simulink model "Model_Composite_2Link_NN_highgain"  (R2019a)
settings: Solver=ode45  StartTime=0.0  StopTime=25  FixedStep=0.0001  RelTol=1e-6  EnableMultiTasking=on
values from neighbouring files (symbols this model uses):
  alpha = 10    [Sim6_highgain.m]
  k = 50    [Sim6_highgain.m]
  kn = 10    [Sim6_highgain.m]
  ks = 1    [Sim6_highgain.m]
  proj1 = 4.5    [Sim6_highgain.m]
  proj2 = 6.7    [Sim6_highgain.m]
  v_initial = zeros(7,5)    [Sim6_highgain.m]
  w_initial = zeros(6,2)    [Sim6_highgain.m]
undefined symbols (not defined in the file or in its folder): gamma1, gamma2
settings Model: Creator=Tenghu  LastModifiedBy=normal
settings DataIOCC: SaveFormat=Array  SignalLoggingSaveFormat=ModelDataLogs  ReturnWorkspaceOutputs=off
settings OptimizationCC: ExpressionDepthLimit=2147483647  EfficientMapNaN2IntZero=off  LifeSpan=inf
settings DebuggingCC: UnderspecifiedInitializationDetection=Classic  MergeDetectMultiDrivingBlocksExec=none  FcnCallInpInsideContextMsg=warning  StateNameClashWarn=warning  SFUnexpectedBacktrackingDiag=warning  SFNoUnconditionalDefaultTransitionDiag=warning  SFExecutionAtInitializationDiag=none  ArithmeticOperatorsInVariantConditions=warning
settings HardwareCC: ProdBitPerPointer=32  ProdBitPerSizeT=32  ProdBitPerPtrDiffT=32  ProdLargestAtomicFloat=None  ProdIntDivRoundTo=Undefined  ProdEndianess=Unspecified  ProdWordSize=32  ProdHWDeviceType=32-bit Generic  TargetBitPerPointer=64  TargetBitPerSizeT=64  TargetBitPerPtrDiffT=64  TargetLongLongMode=on  TargetIntDivRoundTo=Zero  TargetEndianess=LittleEndian  TargetWordSize=64  TargetHWDeviceType=MATLAB Host  ProdEqTarget=off
settings ModelReferenceCC: PropagateSignalLabelsOutOfModel=off
settings SFSimCC: SimUseLocalCustomCode=off  SimParseCustomCode=off
settings RTWCC: RTWUseLocalCustomCode=off
settings CodeAppCC: MaxIdLength=128  StateflowObjectComments=on
settings GRTTargetCC: TargetLangStandard=C89/C90 (ANSI)  GeneratePreprocessorConditionals=Disable all  CombineOutputUpdateFcns=off  GRTInterface=on
settings ConfigComp: CovMetricSettings=dw  CovHtmlReporting=on  CovSaveCumulativeToWorkspaceVar=on  CovSaveSingleToWorkspaceVar=on  CovExternalEMLEnable=off

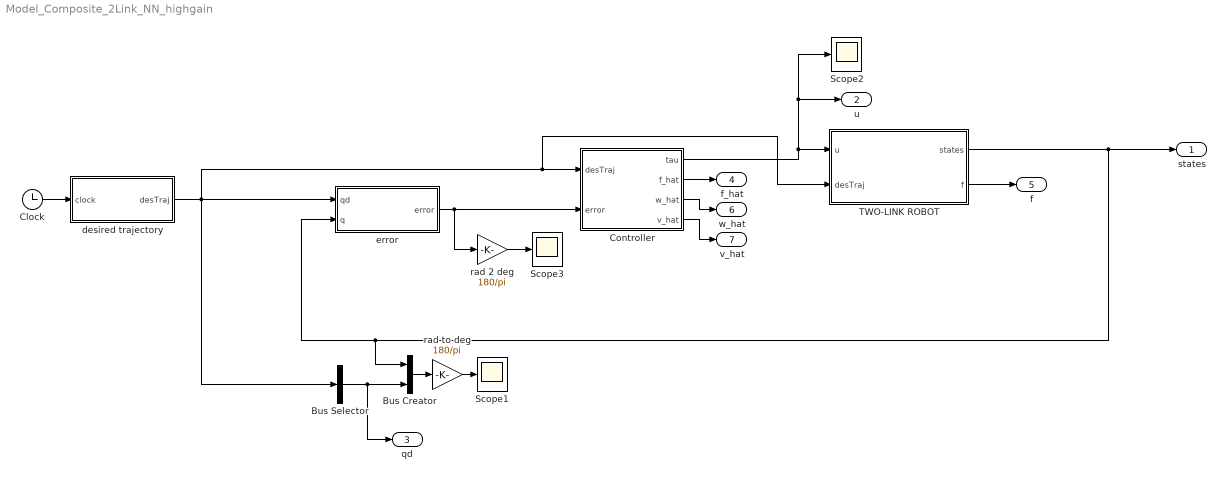
== system Model_Composite_2Link_NN_highgain ==
  Bus Creator : BusCreator  Inputs=2
  Bus Selector : BusSelector  OutputSignals=qd,qdDot  OutputAsBus=on
  Clock : Clock
  Controller : Subsystem
  Scope1 : Scope
  Scope2 : Scope
  Scope3 : Scope
  TWO-LINK ROBOT : Subsystem
  desired trajectory : Subsystem
  error : Subsystem
  rad 2 deg : Gain  Gain=180/pi
  rad to deg : Gain  Gain=180/pi
  states : Outport
  u : Outport  Port=2
  qd : Outport  Port=3
  f_hat : Outport  Port=4
  f : Outport  Port=5
  w_hat : Outport  Port=6
  v_hat : Outport  Port=7
  wires:
  Clock/1 -> desired trajectory/1(clock)
  desired trajectory/1(desTraj) -> error/1(qd), TWO-LINK ROBOT/2(desTraj), Controller/1(desTraj), Bus Selector/1
  rad 2 deg/1 -> Scope3/1
  Bus Creator/1 -> rad to deg/1
  rad to deg/1 -> Scope1/1
  error/1(error) -> Controller/2(error), rad 2 deg/1
  TWO-LINK ROBOT/1(states) -> Bus Creator/1, error/2(q), states/1
  Bus Selector/1 -> qd/1, Bus Creator/2
  Controller/1(tau) -> Scope2/1, u/1, TWO-LINK ROBOT/1(u)
  Controller/2(f_hat) -> f_hat/1
  TWO-LINK ROBOT/2(f) -> f/1
  Controller/3(w_hat) -> w_hat/1
  Controller/4(v_hat) -> v_hat/1

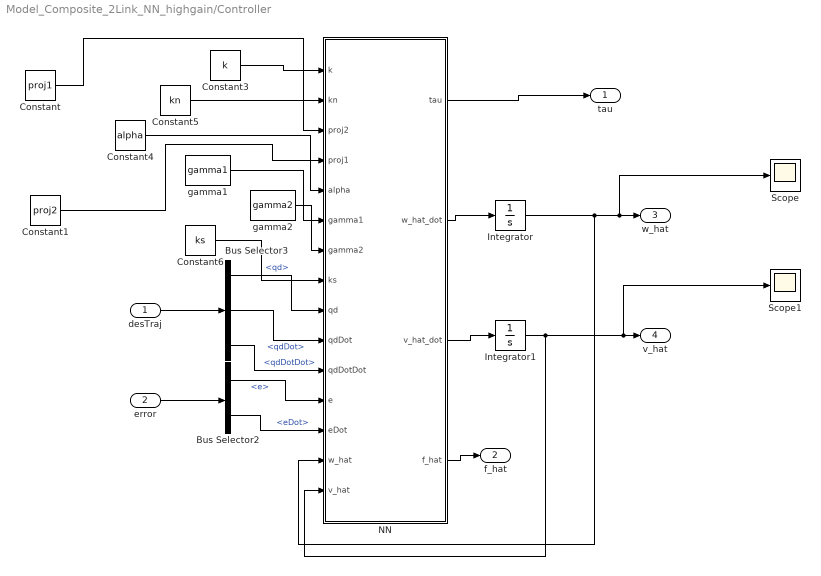
== system Model_Composite_2Link_NN_highgain/Controller ==
  desTraj : Inport
  error : Inport  Port=2
  Bus Selector2 : BusSelector  OutputSignals=e,eDot
  Bus Selector3 : BusSelector  OutputSignals=qd,qdDot,qdDotDot
  Constant : Constant  Value=proj1
  Constant1 : Constant  Value=proj2
  Constant3 : Constant  Value=k
  Constant4 : Constant  Value=alpha
  Constant5 : Constant  Value=kn
  Constant6 : Constant  Value=ks
  Integrator : Integrator  InitialCondition=w_initial
  Integrator1 : Integrator  InitialCondition=v_initial
  NN : MATLAB Function  TreatAsAtomicUnit=on
  Scope : Scope
  Scope1 : Scope
  gamma1 : Constant  Value=gamma1
  gamma2 : Constant  Value=gamma2
  tau : Outport
  f_hat : Outport  Port=2
  w_hat : Outport  Port=3
  v_hat : Outport  Port=4
  wires:
  Bus Selector2/1 -> NN/12(e)  "<e>"
  Bus Selector2/2 -> NN/13(eDot)  "<eDot>"
  error/1 -> Bus Selector2/1
  Bus Selector3/1 -> NN/9(qd)  "<qd>"
  Bus Selector3/3 -> NN/11(qdDotDot)  "<qdDotDot>"
  desTraj/1 -> Bus Selector3/1
  Bus Selector3/2 -> NN/10(qdDot)  "<qdDot>"
  Constant3/1 -> NN/1(k)
  Constant4/1 -> NN/5(alpha)
  Constant5/1 -> NN/2(kn)
  NN/2(w_hat_dot) -> Integrator/1
  NN/3(v_hat_dot) -> Integrator1/1
  Integrator1/1 -> Scope1/1, v_hat/1, NN/15(v_hat)
  Integrator/1 -> Scope/1, w_hat/1, NN/14(w_hat)
  gamma1/1 -> NN/6(gamma1)
  gamma2/1 -> NN/7(gamma2)
  NN/1(tau) -> tau/1
  NN/4(f_hat) -> f_hat/1
  Constant6/1 -> NN/8(ks)
  Constant/1 -> NN/3(proj2)
  Constant1/1 -> NN/4(proj1)

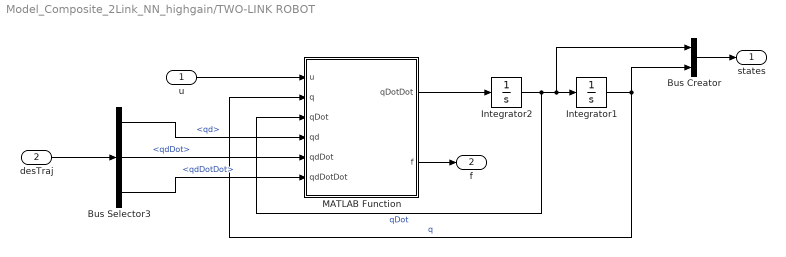
== system Model_Composite_2Link_NN_highgain/TWO-LINK ROBOT ==
  u : Inport
  desTraj : Inport  Port=2
  Bus Creator : BusCreator  Inputs=2
  Bus Selector3 : BusSelector  OutputSignals=qd,qdDot,qdDotDot
  Integrator1 : Integrator  InitialCondition=[0;2]
  Integrator2 : Integrator  InitialCondition=[0;0]
  MATLAB Function : MATLAB Function  TreatAsAtomicUnit=on
  states : Outport
  f : Outport  Port=2
  wires:
  u/1 -> MATLAB Function/1(u)
  Integrator1/1 -> Bus Creator/2, MATLAB Function/2(q)  "q"
  Integrator2/1 -> MATLAB Function/3(qDot), Bus Creator/1, Integrator1/1  "qDot"
  Bus Creator/1 -> states/1
  MATLAB Function/1(qDotDot) -> Integrator2/1
  Bus Selector3/1 -> MATLAB Function/4(qd)  "<qd>"
  Bus Selector3/3 -> MATLAB Function/6(qdDotDot)  "<qdDotDot>"
  desTraj/1 -> Bus Selector3/1
  Bus Selector3/2 -> MATLAB Function/5(qdDot)  "<qdDot>"
  MATLAB Function/2(f) -> f/1

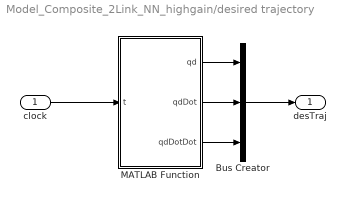
== system Model_Composite_2Link_NN_highgain/desired trajectory ==
  clock : Inport
  Bus Creator : BusCreator  Inputs=3
  MATLAB Function : MATLAB Function  TreatAsAtomicUnit=on
  desTraj : Outport
  wires:
  clock/1 -> MATLAB Function/1(t)
  MATLAB Function/1(qd) -> Bus Creator/1
  MATLAB Function/2(qdDot) -> Bus Creator/2
  MATLAB Function/3(qdDotDot) -> Bus Creator/3
  Bus Creator/1 -> desTraj/1

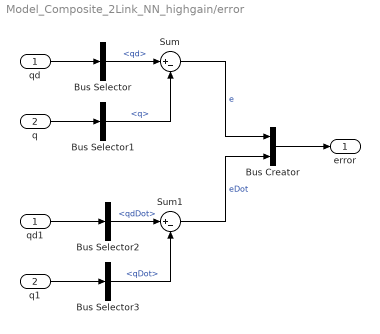
== system Model_Composite_2Link_NN_highgain/error ==
  qd : Inport
  q : Inport  Port=2
  Bus Creator : BusCreator  Inputs=2
  Bus Selector : BusSelector  OutputSignals=qd
  Bus Selector1 : BusSelector  OutputSignals=q
  Bus Selector2 : BusSelector  OutputSignals=qdDot
  Bus Selector3 : BusSelector  OutputSignals=qDot
  Sum : Sum  Inputs=|+-
  Sum1 : Sum  Inputs=|+-
  q1 : InportShadow  Port=2
  qd1 : InportShadow
  error : Outport
  wires:
  qd/1 -> Bus Selector/1
  q/1 -> Bus Selector1/1
  qd1/1 -> Bus Selector2/1
  q1/1 -> Bus Selector3/1
  Bus Selector/1 -> Sum/1  "<qd>"
  Bus Selector1/1 -> Sum/2  "<q>"
  Sum/1 -> Bus Creator/1  "e"
  Bus Selector2/1 -> Sum1/1  "<qdDot>"
  Bus Selector3/1 -> Sum1/2  "<qDot>"
  Bus Creator/1 -> error/1
  Sum1/1 -> Bus Creator/2  "eDot"

== matlab function Model_Composite_2Link_NN_highgain/desired trajectory/MATLAB Function ==
  data: t input; qd output; qdDot output; qdDotDot output
function [qd,qdDot,qdDotDot]  = des_trajectory(t)
%#codegen

% This block supports an embeddable subset of the MATLAB language.
% See the help menu for details. 

qd1=cos(0.5*t);
qd2=2*cos(t);

qd1_dot=-0.5*sin(0.5*t);
qd2_dot=-2*sin(t);

qd1_dotDot = -0.25*cos(0.25*t);
qd2_dotDot = -2*cos(t);

qd=[qd1;qd2];
qdDot = [qd1_dot;qd2_dot];
qdDotDot = [qd1_dotDot; qd2_dotDot];

end

== matlab function Model_Composite_2Link_NN_highgain/Controller/NN ==
  data: k input; kn input; proj2 input; proj1 input; tau output; alpha input; gamma1 input; gamma2 input; ks input; qd input; qdDot input; qdDotDot input; e input; eDot input; w_hat input; v_hat input; w_hat_dot output; v_hat_dot output; f_hat output
function [tau,w_hat_dot,v_hat_dot,f_hat]= controller1(k,kn,proj2, proj1, alpha,gamma1,gamma2,ks,qd,qdDot,qdDotDot,e,eDot,w_hat,v_hat)
%#codegen

q = qd-e; % Check
qDot = qdDot-eDot; % Check
r = eDot+alpha*e; % Check

qd_vec = [1 qd' qdDot' qdDotDot']'; % (7x1)
vq = v_hat'*qd_vec; % (5x7)(7x1) = (5x1)

sigma = exp(-(vq).^2./2); % (5x1)

sigma_vec = [1 sigma']';   % (6x1)
sigma_prime_vec = [1 1 1 1 1; exp(-(vq.^2)./2)*vq'];     %; sigma_prime'; sigma_prime'; sigma_prime'; sigma_prime'; sigma_prime']; % (6x5)

tau = k*r + kn*r + e + w_hat'*sigma_vec ; % (2x6)(6x1)=(2x1)

w_hat_dot = gamma1*sigma_vec*r'; %(6x1)(1x2)=(6x2)
v_hat_dot = gamma2*qd_vec*r'*w_hat'*sigma_prime_vec; %(7x1)(1x2)(2x6)(6x5)=(7x5)

f_hat = w_hat'*sigma_vec; %(2x6)(6x1)=(2x1)

%saturating using projection function
%vHat projection
[v_hat_dot] = Proj(v_hat,v_hat_dot,proj1,-proj1,0.0001);

%w_hat_dot projection function
[w_hat_dot] = Proj(w_hat,w_hat_dot,proj2,-proj2,0.0001);


f_hat = w_hat'*sigma_vec; %(2x6)(6x1)=(2x1)



%projection function definition
function [out] = Proj(theta_hat_curr, theta_hat_dot, upperlim, lowerlim,dt) %functio
[I,J] = size(theta_hat_curr); %initialy matrix definition
out = zeros(I,J);             %initial dummy matrix to be edited later
theta_hat = theta_hat_curr + dt*theta_hat_dot; %proposed update 

% check the proposed update for each index and don't allow it to change
% if it will drive the estimate out of the upper or lower limit
for i = 1:I
    for j = 1:J
        if theta_hat(i,j) >= upperlim && theta_hat_dot(i,j) > 0
            out(i,j) = 0;
        elseif theta_hat(i,j) <= lowerlim && theta_hat_dot(i,j) < 0
            out(i,j) = 0;
        else
            out(i,j) = theta_hat_dot(i,j);
        end
    end
end

end
end

== matlab function Model_Composite_2Link_NN_highgain/TWO-LINK ROBOT/MATLAB Function ==
  data: u input; q input; qDotDot output; qDot input; qd input; qdDot input; qdDotDot input; f output
function [qDotDot,f] = dynamics(u,q,qDot,qd,qdDot,qdDotDot)
%#codegen

p1 = 3.473;
p2 = 0.196;
p3 = 0.242;

fd1 = 5.3;
fd2 = 1.1;

M = [p1+2*p3*cos(q(2)), p2+p3*cos(q(2)); p2+p3*cos(q(2)), p2];
Vm = [-p3*sin(q(2))*qDot(2), -p3*sin(q(2))*(qDot(1)+qDot(2)); p3*sin(q(2))*qDot(1), 0];
Fd = [fd1, 0; 0, fd2];

qDotDot = M\(u - Vm*qDot - Fd*qDot);


M_d = [p1+2*p3*cos(qd(2)), p2+p3*cos(qd(2)); p2+p3*cos(qd(2)), p2];
Vm_d = [-p3*sin(qd(2))*qdDot(2), -p3*sin(qd(2))*(qdDot(1)+qdDot(2)); p3*sin(qd(2))*qdDot(1), 0];
Fd_d = [fd1, 0; 0, fd2];

f = M_d*qdDotDot+Vm_d*qdDot+Fd_d*qdDot;


end
